simulink model "antiwindup_basic_reference"  (R2021a)
settings: Solver=VariableStepAuto  StartTime=0.0  StopTime=1  RelTol=1e-8
settings Model: Creator=cnjones  LastModifiedBy=马骏涛
settings SolverCC: AlgebraicLoopSolver=TrustRegion
settings RTWCC: DLArmComputeVersion=20.02.1

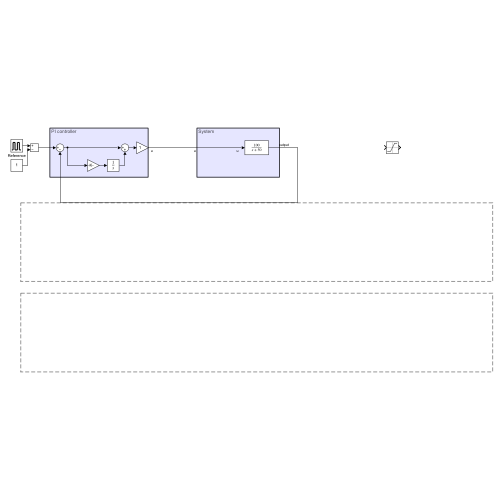
[thumbnail: Simulink's stored preview of the top-level diagram]
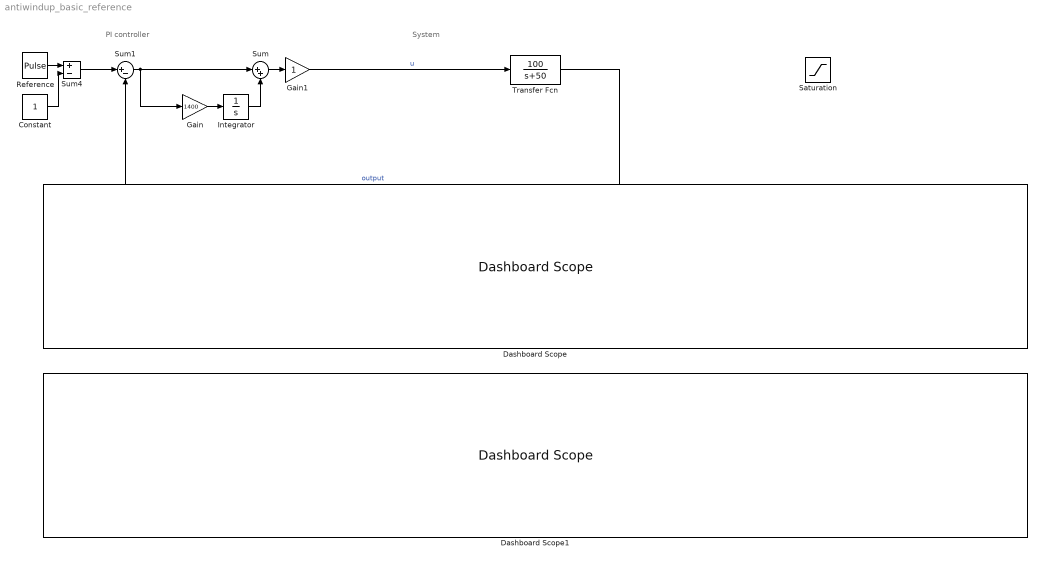
== system antiwindup_basic_reference ==
  note: System
  note: PI controller
  Constant : Constant
  Dashboard Scope : DashboardScope  Ymin=-2  Ymax=2
  Dashboard Scope1 : DashboardScope  Ymin=-1  Ymax=2
  Gain : Gain  Gain=1400
  Gain1 : Gain
  Integrator : Integrator
  Reference : DiscretePulseGenerator  PulseType=Time based  Amplitude=2  Period=0.25  PulseWidth=50
  Saturation : Saturate  UpperLimit=2  LowerLimit=-2
  Sum : Sum  Inputs=|++
  Sum1 : Sum  Inputs=|+-
  Sum4 : Sum  Inputs=+-
  Transfer Fcn : TransferFcn  Numerator=100  Denominator=[1 50]
  wires:
  Gain/1 -> Integrator/1
  Sum/1 -> Gain1/1
  Integrator/1 -> Sum/2
  Transfer Fcn/1 -> Sum1/2  "output"
  Sum1/1 -> Gain/1, Sum/1
  Reference/1 -> Sum4/1
  Constant/1 -> Sum4/2
  Sum4/1 -> Sum1/1
  Gain1/1 -> Transfer Fcn/1  "u"
